simulink model "SAR_logic_organized"  (R2018b)
settings: Solver=VariableStepAuto  StartTime=0.0  StopTime=39  RelTol=1e-3
libraries: simulink_extras x36, simulink x1
settings Model: Creator=iamcy  LastModifiedBy=iamcy

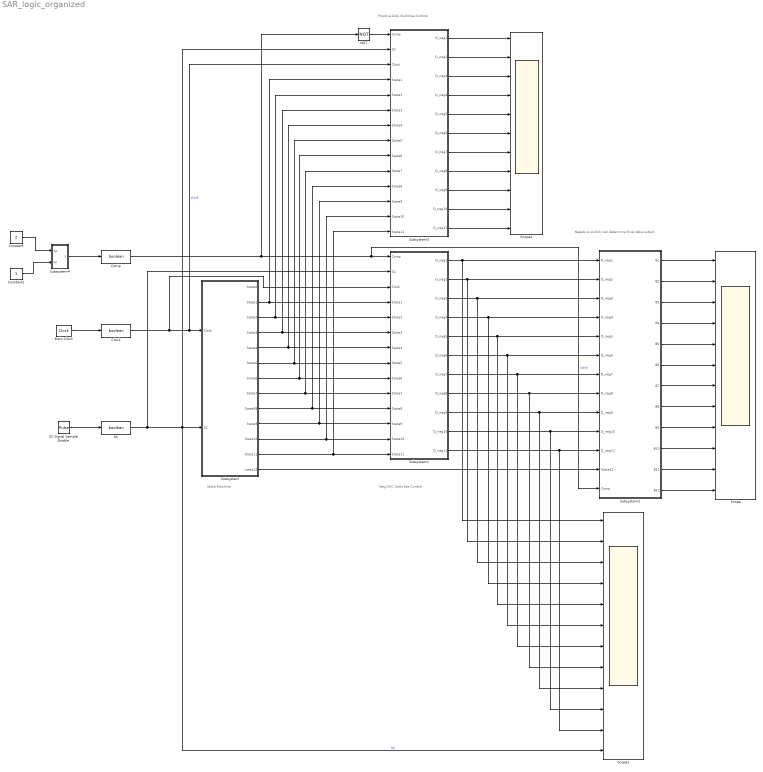
== system SAR_logic_organized ==
  note: Negative switch can determine final data output
  note: Neg DAC Switches Control
  note: State Machine
  note: Positive DAC Switches Control
  Clock : DataTypeConversion  OutDataTypeStr=boolean
  Comp : DataTypeConversion  OutDataTypeStr=boolean
  Constant : Constant  Value=2
  Constant1 : Constant
  Main Clock : simulink_extras/Flip Flops/Clock  period=1
  NOT : Logic  Operator=NOT  IconShape=distinctive  AllPortsSameDT=off  OutDataTypeStr=boolean
  SC : DataTypeConversion  OutDataTypeStr=boolean
  SC Signal Sample Enable : DiscretePulseGenerator  PulseType=Time based  Period=13  PulseWidth=100/13
  Scope : Scope  NumInputPorts=12
  Scope1 : Scope  NumInputPorts=12
  Scope2 : Scope  NumInputPorts=11
  Subsystem : Subsystem
  Subsystem1 : Subsystem
  Subsystem2 : Subsystem
  Subsystem3 : Subsystem
  Subsystem4 : Subsystem
  wires:
  Main Clock/1 -> Clock/1
  SC Signal Sample Enable/1 -> SC/1
  SC/1 -> Subsystem1/2(SC), Scope1/12, Subsystem3/2(SC), Subsystem/2(SC)  "SC"
  Clock/1 -> Subsystem1/3(Clock), Subsystem3/3(Clock), Subsystem/1(Clock)  "clock"
  Subsystem/2(State1) -> Subsystem3/4(State1), Subsystem1/4(State1)
  Subsystem/3(State2) -> Subsystem3/5(State2), Subsystem1/5(State2)
  Subsystem/4(State3) -> Subsystem3/6(State3), Subsystem1/6(State3)
  Subsystem/5(State4) -> Subsystem3/7(State4), Subsystem1/7(State4)
  Subsystem/6(State5) -> Subsystem3/8(State5), Subsystem1/8(State5)
  Subsystem/7(State6) -> Subsystem3/9(State6), Subsystem1/9(State6)
  Subsystem/8(State7) -> Subsystem3/10(State7), Subsystem1/10(State7)
  Subsystem/9(State08) -> Subsystem3/11(State8), Subsystem1/11(State8)
  Subsystem/10(State9) -> Subsystem3/12(State9), Subsystem1/12(State9)
  Subsystem/11(State10) -> Subsystem3/13(State10), Subsystem1/13(State10)
  Subsystem/12(State11) -> Subsystem3/14(State11), Subsystem1/14(State11)
  Subsystem4/1(Comp) -> Comp/1
  Comp/1 -> NOT/1, Subsystem2/13(Comp), Subsystem1/1(Comp)  "clock"
  Subsystem1/1(D_neg1) -> Scope1/1, Subsystem2/1(D_neg1)
  Subsystem1/2(D_neg2) -> Subsystem2/2(D_neg2), Scope1/2
  Subsystem1/3(D_neg3) -> Scope1/3, Subsystem2/3(D_neg3)
  Subsystem1/4(D_neg4) -> Scope1/4, Subsystem2/4(D_neg4)
  Subsystem1/5(D_neg5) -> Subsystem2/5(D_neg5), Scope1/5
  Subsystem1/6(D_neg6) -> Scope1/6, Subsystem2/6(D_neg6)
  Subsystem1/7(D_neg7) -> Scope1/7, Subsystem2/7(D_neg7)
  Subsystem1/8(D_neg8) -> Scope1/8, Subsystem2/8(D_neg8)
  Subsystem1/9(D_neg9) -> Scope1/9, Subsystem2/9(D_neg9)
  Subsystem1/10(D_neg10) -> Scope1/10, Subsystem2/10(D_neg10)
  Subsystem1/11(D_neg11) -> Scope1/11, Subsystem2/11(D_neg11)
  Subsystem/13(state12) -> Subsystem2/12(State12)
  Subsystem2/1(B1) -> Scope/1
  Subsystem2/2(B2) -> Scope/2
  Subsystem2/3(B3) -> Scope/3
  Subsystem2/4(B4) -> Scope/4
  Subsystem2/5(B5) -> Scope/5
  Subsystem2/6(B6) -> Scope/6
  Subsystem2/7(B7) -> Scope/7
  Subsystem2/8(B8) -> Scope/8
  Subsystem2/9(B9) -> Scope/9
  Subsystem2/10(B10) -> Scope/10
  Subsystem2/11(B11) -> Scope/11
  Subsystem2/12(B12) -> Scope/12
  Subsystem3/1(D_neg1) -> Scope2/1
  Subsystem3/2(D_neg2) -> Scope2/2
  Subsystem3/3(D_neg3) -> Scope2/3
  Subsystem3/4(D_neg4) -> Scope2/4
  Subsystem3/5(D_neg5) -> Scope2/5
  Subsystem3/6(D_neg6) -> Scope2/6
  Subsystem3/7(D_neg7) -> Scope2/7
  Subsystem3/8(D_neg8) -> Scope2/8
  Subsystem3/9(D_neg9) -> Scope2/9
  Subsystem3/10(D_neg10) -> Scope2/10
  Subsystem3/11(D_neg11) -> Scope2/11
  NOT/1 -> Subsystem3/1(Comp)
  Constant/1 -> Subsystem4/1(Vp)
  Constant1/1 -> Subsystem4/2(Vn)

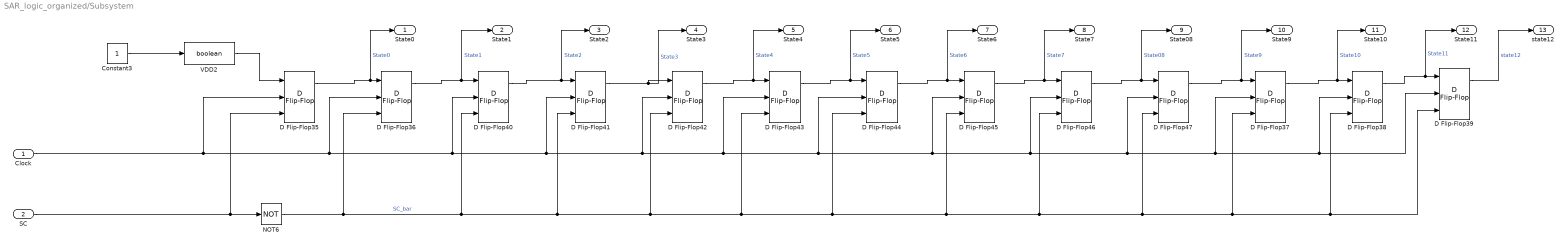
== system SAR_logic_organized/Subsystem ==
  Clock : Inport
  SC : Inport  Port=2
  Constant3 : Constant
  D Flip-Flop{35..47} (13 alike) : simulink_extras/Flip Flops/D Flip-Flop
      settings: SourceProductName=Simulink
  NOT6 : Logic  Operator=NOT  IconShape=distinctive  AllPortsSameDT=off  OutDataTypeStr=boolean
  VDD2 : DataTypeConversion  OutDataTypeStr=boolean
  State0 : Outport
  State1 : Outport  Port=2
  State2 : Outport  Port=3
  State3 : Outport  Port=4
  State4 : Outport  Port=5
  State5 : Outport  Port=6
  State6 : Outport  Port=7
  State7 : Outport  Port=8
  State08 : Outport  Port=9
  State9 : Outport  Port=10
  State10 : Outport  Port=11
  State11 : Outport  Port=12
  state12 : Outport  Port=13
  wires:
  D Flip-Flop43/1 -> State5/1, D Flip-Flop44/1  "State5"
  D Flip-Flop40/1 -> State2/1, D Flip-Flop41/1  "State2"
  D Flip-Flop45/1 -> State7/1, D Flip-Flop46/1  "State7"
  D Flip-Flop38/1 -> State11/1, D Flip-Flop39/1  "State11"
  D Flip-Flop42/1 -> State4/1, D Flip-Flop43/1  "State4"
  D Flip-Flop44/1 -> State6/1, D Flip-Flop45/1  "State6"
  NOT6/1 -> D Flip-Flop42/3, D Flip-Flop44/3, D Flip-Flop46/3, D Flip-Flop38/3, D Flip-Flop39/3, D Flip-Flop37/3, D Flip-Flop47/3, D Flip-Flop45/3, D Flip-Flop43/3, D Flip-Flop41/3, D Flip-Flop40/3, D Flip-Flop36/3  "SC_bar"
  D Flip-Flop36/1 -> State1/1, D Flip-Flop40/1  "State1"
  Clock/1 -> D Flip-Flop36/2, D Flip-Flop41/2, D Flip-Flop42/2, D Flip-Flop43/2, D Flip-Flop44/2, D Flip-Flop45/2, D Flip-Flop46/2, D Flip-Flop38/2, D Flip-Flop39/2, D Flip-Flop37/2, D Flip-Flop47/2, D Flip-Flop40/2, D Flip-Flop35/2
  D Flip-Flop47/1 -> State9/1, D Flip-Flop37/1  "State9"
  Constant3/1 -> VDD2/1
  D Flip-Flop41/1 -> State3/1, D Flip-Flop42/1  "State3"
  D Flip-Flop37/1 -> State10/1, D Flip-Flop38/1  "State10"
  D Flip-Flop35/1 -> State0/1, D Flip-Flop36/1  "State0"
  D Flip-Flop46/1 -> State08/1, D Flip-Flop47/1  "State08"
  SC/1 -> NOT6/1, D Flip-Flop35/3
  VDD2/1 -> D Flip-Flop35/1
  D Flip-Flop39/1 -> state12/1  "state12"

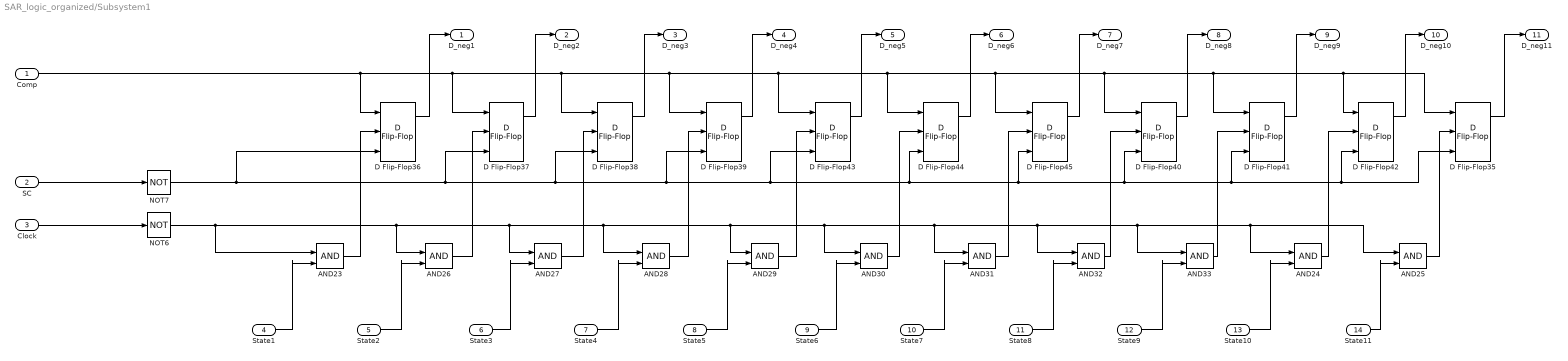
== system SAR_logic_organized/Subsystem1 ==
  Comp : Inport
  SC : Inport  Port=2
  Clock : Inport  Port=3
  State1 : Inport  Port=4
  State2 : Inport  Port=5
  State3 : Inport  Port=6
  State4 : Inport  Port=7
  State5 : Inport  Port=8
  State6 : Inport  Port=9
  State7 : Inport  Port=10
  State8 : Inport  Port=11
  State9 : Inport  Port=12
  State10 : Inport  Port=13
  State11 : Inport  Port=14
  AND{23..33} (11 alike) : Logic  IconShape=distinctive  AllPortsSameDT=off  OutDataTypeStr=boolean
  D Flip-Flop{35..45} (11 alike) : simulink_extras/Flip Flops/D Flip-Flop
      settings: SourceProductName=Simulink
  NOT6 : Logic  Operator=NOT  IconShape=distinctive  AllPortsSameDT=off  OutDataTypeStr=boolean
  NOT7 : Logic  Operator=NOT  IconShape=distinctive  AllPortsSameDT=off  OutDataTypeStr=boolean
  D_neg1 : Outport
  D_neg2 : Outport  Port=2
  D_neg3 : Outport  Port=3
  D_neg4 : Outport  Port=4
  D_neg5 : Outport  Port=5
  D_neg6 : Outport  Port=6
  D_neg7 : Outport  Port=7
  D_neg8 : Outport  Port=8
  D_neg9 : Outport  Port=9
  D_neg10 : Outport  Port=10
  D_neg11 : Outport  Port=11
  wires:
  NOT7/1 -> D Flip-Flop35/3, D Flip-Flop42/3, D Flip-Flop41/3, D Flip-Flop40/3, D Flip-Flop45/3, D Flip-Flop44/3, D Flip-Flop43/3, D Flip-Flop39/3, D Flip-Flop38/3, D Flip-Flop37/3, D Flip-Flop36/3
  D Flip-Flop41/1 -> D_neg9/1
  AND23/1 -> D Flip-Flop36/2
  State9/1 -> AND33/2
  Comp/1 -> D Flip-Flop35/1, D Flip-Flop42/1, D Flip-Flop41/1, D Flip-Flop40/1, D Flip-Flop45/1, D Flip-Flop44/1, D Flip-Flop43/1, D Flip-Flop39/1, D Flip-Flop38/1, D Flip-Flop37/1, D Flip-Flop36/1
  D Flip-Flop42/1 -> D_neg10/1
  AND27/1 -> D Flip-Flop38/2
  NOT6/1 -> AND25/1, AND24/1, AND33/1, AND32/1, AND31/1, AND30/1, AND29/1, AND28/1, AND27/1, AND26/1, AND23/1
  AND25/1 -> D Flip-Flop35/2
  AND29/1 -> D Flip-Flop43/2
  AND31/1 -> D Flip-Flop45/2
  AND28/1 -> D Flip-Flop39/2
  State1/1 -> AND23/2
  AND33/1 -> D Flip-Flop41/2
  D Flip-Flop45/1 -> D_neg7/1
  State5/1 -> AND29/2
  AND26/1 -> D Flip-Flop37/2
  AND24/1 -> D Flip-Flop42/2
  SC/1 -> NOT7/1
  AND32/1 -> D Flip-Flop40/2
  State10/1 -> AND24/2
  AND30/1 -> D Flip-Flop44/2
  D Flip-Flop38/1 -> D_neg3/1
  Clock/1 -> NOT6/1
  D Flip-Flop36/1 -> D_neg1/1
  D Flip-Flop37/1 -> D_neg2/1
  D Flip-Flop35/1 -> D_neg11/1
  D Flip-Flop43/1 -> D_neg5/1
  State4/1 -> AND28/2
  State3/1 -> AND27/2
  State2/1 -> AND26/2
  State8/1 -> AND32/2
  D Flip-Flop44/1 -> D_neg6/1
  State6/1 -> AND30/2
  State11/1 -> AND25/2
  D Flip-Flop40/1 -> D_neg8/1
  State7/1 -> AND31/2
  D Flip-Flop39/1 -> D_neg4/1

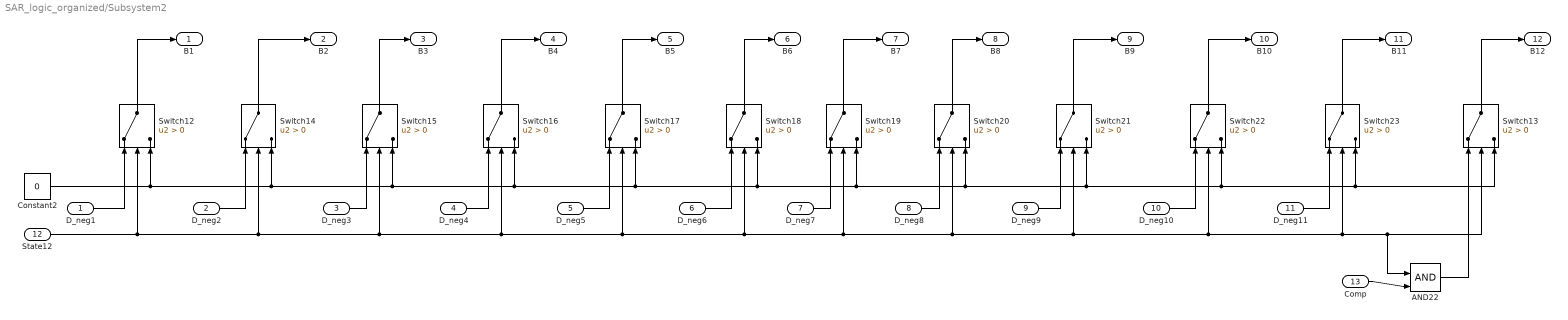
== system SAR_logic_organized/Subsystem2 ==
  D_neg1 : Inport
  D_neg2 : Inport  Port=2
  D_neg3 : Inport  Port=3
  D_neg4 : Inport  Port=4
  D_neg5 : Inport  Port=5
  D_neg6 : Inport  Port=6
  D_neg7 : Inport  Port=7
  D_neg8 : Inport  Port=8
  D_neg9 : Inport  Port=9
  D_neg10 : Inport  Port=10
  D_neg11 : Inport  Port=11
  State12 : Inport  Port=12
  Comp : Inport  Port=13
  AND22 : Logic  IconShape=distinctive  AllPortsSameDT=off  OutDataTypeStr=boolean
  Constant2 : Constant  Value=0
  Switch{12..23} (12 alike) : Switch  Criteria=u2 > Threshold
  B1 : Outport
  B2 : Outport  Port=2
  B3 : Outport  Port=3
  B4 : Outport  Port=4
  B5 : Outport  Port=5
  B6 : Outport  Port=6
  B7 : Outport  Port=7
  B8 : Outport  Port=8
  B9 : Outport  Port=9
  B10 : Outport  Port=10
  B11 : Outport  Port=11
  B12 : Outport  Port=12
  wires:
  Constant2/1 -> Switch12/3, Switch13/3, Switch23/3, Switch22/3, Switch21/3, Switch20/3, Switch19/3, Switch18/3, Switch17/3, Switch16/3, Switch15/3, Switch14/3
  Switch22/1 -> B10/1
  Switch17/1 -> B5/1
  Switch12/1 -> B1/1
  Switch14/1 -> B2/1
  Switch18/1 -> B6/1
  Switch16/1 -> B4/1
  Switch15/1 -> B3/1
  Switch23/1 -> B11/1
  Switch20/1 -> B8/1
  Switch21/1 -> B9/1
  Switch19/1 -> B7/1
  Switch13/1 -> B12/1
  State12/1 -> Switch12/2, Switch14/2, Switch15/2, Switch16/2, Switch17/2, Switch19/2, Switch20/2, Switch21/2, Switch22/2, AND22/1, Switch13/2, Switch23/2, Switch18/2
  AND22/1 -> Switch13/1
  Comp/1 -> AND22/2
  D_neg11/1 -> Switch23/1
  D_neg10/1 -> Switch22/1
  D_neg9/1 -> Switch21/1
  D_neg8/1 -> Switch20/1
  D_neg7/1 -> Switch19/1
  D_neg6/1 -> Switch18/1
  D_neg5/1 -> Switch17/1
  D_neg4/1 -> Switch16/1
  D_neg3/1 -> Switch15/1
  D_neg2/1 -> Switch14/1
  D_neg1/1 -> Switch12/1

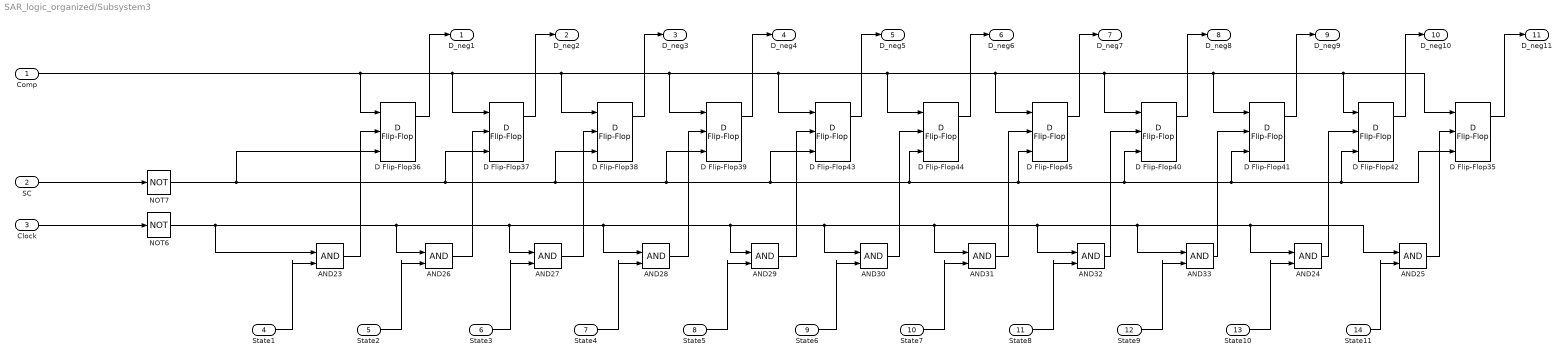
== system SAR_logic_organized/Subsystem3 ==
  Comp : Inport
  SC : Inport  Port=2
  Clock : Inport  Port=3
  State1 : Inport  Port=4
  State2 : Inport  Port=5
  State3 : Inport  Port=6
  State4 : Inport  Port=7
  State5 : Inport  Port=8
  State6 : Inport  Port=9
  State7 : Inport  Port=10
  State8 : Inport  Port=11
  State9 : Inport  Port=12
  State10 : Inport  Port=13
  State11 : Inport  Port=14
  AND{23..33} (11 alike) : Logic  IconShape=distinctive  AllPortsSameDT=off  OutDataTypeStr=boolean
  D Flip-Flop{35..45} (11 alike) : simulink_extras/Flip Flops/D Flip-Flop
      settings: SourceProductName=Simulink
  NOT6 : Logic  Operator=NOT  IconShape=distinctive  AllPortsSameDT=off  OutDataTypeStr=boolean
  NOT7 : Logic  Operator=NOT  IconShape=distinctive  AllPortsSameDT=off  OutDataTypeStr=boolean
  D_neg1 : Outport
  D_neg2 : Outport  Port=2
  D_neg3 : Outport  Port=3
  D_neg4 : Outport  Port=4
  D_neg5 : Outport  Port=5
  D_neg6 : Outport  Port=6
  D_neg7 : Outport  Port=7
  D_neg8 : Outport  Port=8
  D_neg9 : Outport  Port=9
  D_neg10 : Outport  Port=10
  D_neg11 : Outport  Port=11
  wires:
  NOT7/1 -> D Flip-Flop35/3, D Flip-Flop42/3, D Flip-Flop41/3, D Flip-Flop40/3, D Flip-Flop45/3, D Flip-Flop44/3, D Flip-Flop43/3, D Flip-Flop39/3, D Flip-Flop38/3, D Flip-Flop37/3, D Flip-Flop36/3
  D Flip-Flop41/1 -> D_neg9/1
  AND23/1 -> D Flip-Flop36/2
  State9/1 -> AND33/2
  Comp/1 -> D Flip-Flop35/1, D Flip-Flop42/1, D Flip-Flop41/1, D Flip-Flop40/1, D Flip-Flop45/1, D Flip-Flop44/1, D Flip-Flop43/1, D Flip-Flop39/1, D Flip-Flop38/1, D Flip-Flop37/1, D Flip-Flop36/1
  D Flip-Flop42/1 -> D_neg10/1
  AND27/1 -> D Flip-Flop38/2
  NOT6/1 -> AND25/1, AND24/1, AND33/1, AND32/1, AND31/1, AND30/1, AND29/1, AND28/1, AND27/1, AND26/1, AND23/1
  AND25/1 -> D Flip-Flop35/2
  AND29/1 -> D Flip-Flop43/2
  AND31/1 -> D Flip-Flop45/2
  AND28/1 -> D Flip-Flop39/2
  State1/1 -> AND23/2
  AND33/1 -> D Flip-Flop41/2
  D Flip-Flop45/1 -> D_neg7/1
  State5/1 -> AND29/2
  AND26/1 -> D Flip-Flop37/2
  AND24/1 -> D Flip-Flop42/2
  SC/1 -> NOT7/1
  AND32/1 -> D Flip-Flop40/2
  State10/1 -> AND24/2
  AND30/1 -> D Flip-Flop44/2
  D Flip-Flop38/1 -> D_neg3/1
  Clock/1 -> NOT6/1
  D Flip-Flop36/1 -> D_neg1/1
  D Flip-Flop37/1 -> D_neg2/1
  D Flip-Flop35/1 -> D_neg11/1
  D Flip-Flop43/1 -> D_neg5/1
  State4/1 -> AND28/2
  State3/1 -> AND27/2
  State2/1 -> AND26/2
  State8/1 -> AND32/2
  D Flip-Flop44/1 -> D_neg6/1
  State6/1 -> AND30/2
  State11/1 -> AND25/2
  D Flip-Flop40/1 -> D_neg8/1
  State7/1 -> AND31/2
  D Flip-Flop39/1 -> D_neg4/1

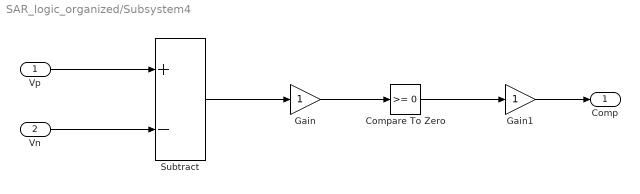
== system SAR_logic_organized/Subsystem4 ==
  Vp : Inport
  Vn : Inport  Port=2
  Compare To Zero : simulink/Logic and Bit Operations/Compare To Zero  relop=>=  OutDataTypeStr=boolean
  Gain : Gain
  Gain1 : Gain
  Subtract : Sum  Inputs=+-
  Comp : Outport
  wires:
  Gain1/1 -> Comp/1
  Subtract/1 -> Gain/1
  Gain/1 -> Compare To Zero/1
  Compare To Zero/1 -> Gain1/1
  Vn/1 -> Subtract/2
  Vp/1 -> Subtract/1
